simulink model "Battery_model_2D_Battery2"  (R2026a)
settings: Solver=VariableStepAuto  StopTime=10000
InitFcn:
  | %% Universal Parameters
  | 
  | Cycle_num = 1000; % number of cycles
  | 
  | Temp_state = 35;
  | 
  | 
  | SoC_state = 0.5;
  | 
  | OCV = [ 3.0025,3.4635,3.521,3.5618,3.6058,3.6426,3.6725,3.7049,3.7486,3.79951,3.8418,3.8738 ,3.9044,3.9448,3.9813,4.0222 ,4.0498,4.0658,4.0919,4.1359,4.2];
  | 
  | 
  | % Cn = 540; % As
  | Ru = 3.19; % KW^-1
  | Rc = 1.94; % KW^-1
  | Cc = 62.7; % JK^-1
  | Cs = 4.5;  % JK^-1
  | 
  | Ea = 31500;  % J * mol^-1
  | eta = 152.5; % unitless
  | Ic = 9000;   % [1/s] normalized current rate
  | Rg = 8.314;  % J / K / mol
  | z = 0.57;    % Ah power law exponent
  | 
  | 
  | 
  | %% Breakpoints
  | Temp = [5, 15, 25, 35, 45];
  | SoC  = [0, 0.05, 0.10, 0.15, 0.20, 0.25, 0.30, 0.35, 0.40, 0.45, 0.50, 0.55, 0.60, 0.65, 0.70, 0.75, 0.80, 0.85, 0.90, 0.95, 1.00];
  | 
  | %% ── CHARGING Parameters ──────────────────────────────────────────────────────
  | %% CHARGING Parameters
  | 
  | % --- R0 (charge) ---
  | R0_5_ch  = [0.10039366, 0.10039366, 0.10039366, 0.08528700, 0.07769698, 0.08283688, 0.11006698 ...
  |              0.11427069, 0.11402639, 0.11444591, 0.11423324, 0.11397462, 0.11400530, 0.11412006 ...
  |              0.11437022, 0.11469884, 0.11501972, 0.11491341, 0.11445199, 0.11423824, 0.11366247];
  | R0_15_ch  = [0.13171649, 0.13171649, 0.13171649, 0.11189655, 0.10193844, 0.10868199, 0.14440788 ...
  |              0.14992315, 0.14960263, 0.15015303, 0.14987401, 0.14953470, 0.14957496, 0.14972552 ...
  |              0.15005372, 0.15048488, 0.15090588, 0.15076639, 0.15016101, 0.14988057, 0.14912516];
  | R0_25_ch  = [0.15680534, 0.15680534, 0.15680534, 0.13321018, 0.12135528, 0.12938332, 0.17191415 ...
  |              0.17847994, 0.17809836, 0.17875361, 0.17842144, 0.17801751, 0.17806543, 0.17824467 ...
  |              0.17863539, 0.17914866, 0.17964985, 0.17948380, 0.17876310, 0.17842925, 0.17752995];
  | R0_35_ch  = [0.18293956, 0.18293956, 0.18293956, 0.15541187, 0.14158117, 0.15094720, 0.20056650 ...
  |              0.20822660, 0.20778142, 0.20854588, 0.20815835, 0.20768709, 0.20774300, 0.20795212 ...
  |              0.20840795, 0.20900677, 0.20959150, 0.20939777, 0.20855695, 0.20816746, 0.20711828];
  | R0_45_ch  = [0.20580701, 0.20580701, 0.20580701, 0.17483836, 0.15927881, 0.16981560, 0.22563732 ...
  |              0.23425492, 0.23375410, 0.23461411, 0.23417814, 0.23364798, 0.23371087, 0.23394613 ...
  |              0.23445894, 0.23513262, 0.23579043, 0.23557249, 0.23462657, 0.23418839, 0.23300807];
  | R0_ch = [R0_5_ch; R0_15_ch; R0_25_ch; R0_35_ch; R0_45_ch];
  | 
  | % --- R1 (charge) ---
  | R1_5_ch  = [0.04985788, 0.04985788, 0.05071229, 0.04160410, 0.03661133, 0.03925367, 0.05381930 ...
  |              0.05642225, 0.05603500, 0.05496214, 0.05471562, 0.05430091, 0.05382478, 0.05367572 ...
  |              0.05355262, 0.05341750, 0.05337771, 0.05361159, 0.05382278, 0.05411150, 0.05453301];
  | R1_15_ch  = [0.07380278, 0.07380278, 0.07506754, 0.06158502, 0.05419440, 0.05810577, 0.07966673 ...
  |              0.08351978, 0.08294655, 0.08135843, 0.08099351, 0.08037963, 0.07967483, 0.07945418 ...
  |              0.07927196, 0.07907196, 0.07901306, 0.07935925, 0.07967188, 0.08009926, 0.08072321];
  | R1_25_ch  = [0.09348353, 0.09348353, 0.09508555, 0.07800769, 0.06864625, 0.07360064, 0.10091119 ...
  |              0.10579172, 0.10506563, 0.10305401, 0.10259178, 0.10181420, 0.10092146, 0.10064197 ...
  | ... (+154 lines)
model workspace (MAT data in the model file):
  C_As = 150
  Cn = 150
  I_c = 1
  I_c_full_charged = 0.0333333333333
  Tc_state = 35.0044118318
  Ts_state = 35.0027406087
  V1_state = 0.00398713164124
  V2_state = 0.00927212980774
  V_cutoff = 3
  V_max = 4.2
  current_SoC = 0.996576803874
undefined symbols (not defined in the file): V1_ini
libraries: simulink x7
(part 2 of 2)

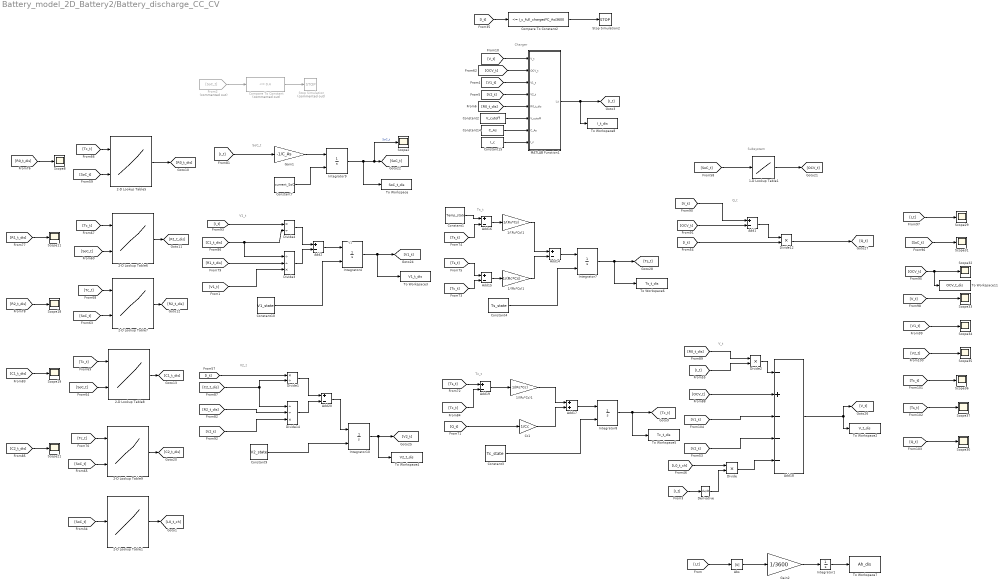
== system Battery_model_2D_Battery2/Battery_discharge_CC_CV ==
  note: Q_t
  note: V1
  note: SoC_t
  note: V1_t
  note: V2_t
  note: V_t
  note: Ts_t
  note: Tc_t
  note: Subsystem
  note: Charger
  1-D Lookup Table1 : Lookup_n-D  NumberOfTableDimensions=1  BreakpointsForDimension1=SoC  BreakpointsForDimension2=Temp  Table=OCV  InternalRulePriority=Speed  RndMeth=Simplest
  1/(Rc*Cc)1 : Gain  Gain=1/(Rc*Cc)
  1/(Rc*Cs)1 : Gain  Gain=1/(Rc*Cs)
  1/(Ru*Cs)1 : Gain  Gain=1/(Ru*Cs)
  2-D Lookup Table1 : Lookup_n-D  NumberOfTableDimensions=1  BreakpointsForDimension1=Temp  BreakpointsForDimension2=SoC  Table=C2_ch  InternalRulePriority=Speed  RndMeth=Simplest
  2-D Lookup Table5 : Lookup_n-D  BreakpointsForDimension1=Temp  BreakpointsForDimension2=SoC  Table=R0_dis  InternalRulePriority=Speed  RndMeth=Simplest
      settings: InputPortMap=u0,u1
  2-D Lookup Table6 : Lookup_n-D  BreakpointsForDimension1=Temp  BreakpointsForDimension2=SoC  Table=R1_dis  InternalRulePriority=Speed  RndMeth=Simplest
      settings: InputPortMap=u0,u1
  2-D Lookup Table7 : Lookup_n-D  BreakpointsForDimension1=Temp  BreakpointsForDimension2=SoC  Table=R2_dis  InternalRulePriority=Speed  RndMeth=Simplest
      settings: InputPortMap=u0,u1
  2-D Lookup Table8 : Lookup_n-D  BreakpointsForDimension1=Temp  BreakpointsForDimension2=SoC  Table=C1_dis  InternalRulePriority=Speed  RndMeth=Simplest
      settings: InputPortMap=u0,u1
  2-D Lookup Table9 : Lookup_n-D  BreakpointsForDimension1=Temp  BreakpointsForDimension2=SoC  Table=C2_dis  InternalRulePriority=Speed  RndMeth=Simplest
      settings: InputPortMap=u0,u1
  Abs : Abs  SaturateOnIntegerOverflow=off
  Add{1..2,14..16,19..20} (7 alike) : Sum  Inputs=+-
  Add17 : Sum
  Add18 : Sum  Inputs=-+---
  Cc1 : Gain  Gain=1/Cc
  Compare To Constant : simulink/Logic and Bit Operations/Compare To Constant  Commented=on  relop=<=  const=0.4  OutDataTypeStr=boolean
  Compare To Constant2 : simulink/Logic and Bit Operations/Compare To Constant  relop=<=  const=I_c_full_charged*C_As/3600  OutDataTypeStr=boolean
  Constant1 : Constant  Value=Temp_state
  Constant10 : Constant  Value=V1_state
  Constant14 : Constant  Value=C_As
  Constant15 : Constant  Value=I_c
  Constant2 : Constant  Value=V_cutoff
  Constant3 : Constant  Value=Tc_state
  Constant4 : Constant  Value=Ts_state
  Constant7 : Constant  Value=current_SoC
  Constant9 : Constant  Value=V2_state
  Derivative : Derivative
  Divide : Product  Inputs=**
  Divide1 : Product  Inputs=*/
  Divide12 : Product  Inputs=**
  Divide14 : Product  Inputs=//*
  Divide2 : Product  Inputs=**
  Divide3 : Product  Inputs=//*
  Divide4 : Product  Inputs=*/
  From2 : From  Commented=on  GotoTag=SoC_t
  Gain1 : Gain  Gain=-1/C_As
  Gain2 : Gain  Gain=1/3600
  Integrator1 : Integrator
  Integrator{4,7..8,10} (4 alike) : Integrator  InitialConditionSource=external
  Integrator9 : Integrator  InitialConditionSource=external  InitialCondition=V1_ini
  MATLAB Function1 : MATLAB Function  TreatAsAtomicUnit=on
  Scope{2,8,11,18..19,21,29..37} (15 alike) : Scope
      Scope11 settings: ActiveDisplayYMinimum=-0.125  ActiveDisplayYMaximum=1.125  DataLoggingVariableName=ScopeData7
      Scope18 settings: ActiveDisplayYMinimum=-0.125  ActiveDisplayYMaximum=1.125  DataLoggingVariableName=ScopeData8
      Scope19 settings: ActiveDisplayYMinimum=-0.125  ActiveDisplayYMaximum=1.125  DataLoggingVariableName=ScopeData9
      Scope2 settings: ActiveDisplayYMinimum=-1  ActiveDisplayYMaximum=1
      Scope21 settings: ActiveDisplayYMinimum=-0.125  ActiveDisplayYMaximum=1.125  DataLoggingVariableName=ScopeData10
      Scope29 settings: ActiveDisplayYMinimum=-0.013121  ActiveDisplayYMaximum=0.16808  DataLoggingVariableName=ScopeData15
      Scope30 settings: ActiveDisplayYMinimum=-0.17004  ActiveDisplayYMaximum=1.5304  DataLoggingVariableName=ScopeData23
      Scope31 settings: ActiveDisplayYMinimum=0.00061627  ActiveDisplayYMaximum=0.00083875  DataLoggingVariableName=ScopeData16
      Scope32 settings: ActiveDisplayYMinimum=2.011  ActiveDisplayYMaximum=4.011  DataLoggingVariableName=ScopeData17
      Scope33 settings: ActiveDisplayYMinimum=2.85  ActiveDisplayYMaximum=3.15  DataLoggingVariableName=ScopeData18
      Scope34 settings: ActiveDisplayYMinimum=0.0016856  ActiveDisplayYMaximum=0.0018374  DataLoggingVariableName=ScopeData19
      Scope35 settings: ActiveDisplayYMinimum=0.006752  ActiveDisplayYMaximum=0.008752  DataLoggingVariableName=ScopeData20
      Scope36 settings: ActiveDisplayYMinimum=-4.1824  ActiveDisplayYMaximum=42.6414  DataLoggingVariableName=ScopeData21
      Scope37 settings: ActiveDisplayYMinimum=2.2586  ActiveDisplayYMaximum=3.6824  DataLoggingVariableName=ScopeData22
      Scope8 settings: ActiveDisplayYMinimum=-0.125  ActiveDisplayYMaximum=1.125  DataLoggingVariableName=ScopeData6
  Stop Simulation : Stop  Commented=on
  Stop Simulation2 : Stop
  To Workspace : ToWorkspace  VariableName=SoC_t_dis  SampleTime=-1
      settings: Save2DSignal=2-D array (concatenate along first dimension)
  To Workspace11 : ToWorkspace  VariableName=OCV_t_dis  SaveFormat=Timeseries  SampleTime=-1
  To Workspace2 : ToWorkspace  VariableName=V_t_dis  SaveFormat=Timeseries  SampleTime=-1
  To Workspace3 : ToWorkspace  VariableName=V1_t_dis  SampleTime=-1
      settings: Save2DSignal=2-D array (concatenate along first dimension)
  To Workspace4 : ToWorkspace  VariableName=V2_t_dis  SampleTime=-1
      settings: Save2DSignal=2-D array (concatenate along first dimension)
  To Workspace5 : ToWorkspace  VariableName=Tc_t_dis  SampleTime=-1
      settings: Save2DSignal=2-D array (concatenate along first dimension)
  To Workspace6 : ToWorkspace  VariableName=Ts_t_dis  SampleTime=-1
      settings: Save2DSignal=2-D array (concatenate along first dimension)
  To Workspace7 : ToWorkspace  VariableName=Ah_dis  SampleTime=-1
      settings: Save2DSignal=2-D array (concatenate along first dimension)
  To Workspace8 : ToWorkspace  VariableName=I_t_dis  SaveFormat=Timeseries  SampleTime=-1
  wires:
  2-D Lookup Table9/1 -> [C2_t_dis]
  [SoC_t] -> 2-D Lookup Table9/2
  Add18/1 -> [V_t], To Workspace2/1
  [V2_t] -> Scope35/1
  Cc1/1 -> Add17/2
  Divide1/1 -> Add20/1
  1-D Lookup Table1/1 -> [OCV_t]
  [SoC_t] -> Scope31/1
  Gain1/1 -> Integrator9/1
  [Tc_t] -> 2-D Lookup Table5/1
  [OCV_t] -> Add18/2
  Integrator10/1 -> To Workspace4/1, [V2_t]
  1/(Rc*Cc)1/1 -> Add17/1
  [R0_t_dis] -> Scope8/1
  Integrator4/1 -> To Workspace3/1, [V1_t]
  Divide4/1 -> Add2/1
  [Ts_t] -> Add19/1
  [C2_t_dis] -> Divide14/1, Divide1/2
  [V2_t] -> Divide14/3
  1/(Ru*Cs)1/1 -> Add14/1
  [SoC_t] -> 2-D Lookup Table8/2
  Add17/1 -> Integrator8/1
  [Tc_t] -> Scope36/1
  Constant1/1 -> Add16/1
  Divide12/1 -> [Q_t]
  2-D Lookup Table8/1 -> [C1_t_dis]
  Integrator7/1 -> To Workspace6/1, [Ts_t]
  1/(Rc*Cs)1/1 -> Add14/2
  [R1_t_dis] -> Scope11/1
  [Ts_t] -> Add16/2
  [V1_t] -> Add18/3
  Add16/1 -> 1/(Ru*Cs)1/1
  Add1/1 -> Divide12/1
  [I_t] -> Scope29/1
  Divide14/1 -> Add20/2
  [R2_t_dis] -> Divide14/2
  [Q_t] -> Scope30/1
  Add14/1 -> Integrator7/1
  Add2/1 -> Integrator4/1
  [Tc_t] -> 2-D Lookup Table7/1
  [V1_t] -> Scope34/1
  2-D Lookup Table7/1 -> [R2_t_dis]
  2-D Lookup Table6/1 -> [R1_t_dis]
  [V2_t] -> Add18/4
  [SoC_t] -> 2-D Lookup Table6/2
  [R2_t_dis] -> Scope18/1
  [SoC_t] -> 2-D Lookup Table5/2
  2-D Lookup Table5/1 -> [R0_t_dis]
  [OCV_t] -> To Workspace11/1, Scope32/1
  [Q_t] -> Cc1/1
  Divide3/1 -> Add2/2
  [I_t] -> Divide12/2
  Add19/1 -> 1/(Rc*Cc)1/1
  Add20/1 -> Integrator10/1
  [C1_t_dis] -> Scope19/1
  Divide2/1 -> Add18/1
  Add15/1 -> 1/(Rc*Cs)1/1
  [R1_t_dis] -> Divide3/2
  [C1_t_dis] -> Divide4/2, Divide3/1
  Integrator9/1 -> To Workspace/1, Scope2/1, [SoC_t]  "SoC_t"
  [Tc_t] -> Add15/2
  [OCV_t] -> Add1/2
  [C2_t_dis] -> Scope21/1
  [Tc_t] -> 2-D Lookup Table8/1
  [V1_t] -> Divide3/3
  [Tc_t] -> 2-D Lookup Table9/1
  [Ts_t] -> Add15/1
  [Ts_t] -> Scope37/1
  [V_t] -> Scope33/1
  [SoC_t] -> 1-D Lookup Table1/1
  [SoC_t] -> 2-D Lookup Table7/2
  [Tc_t] -> 2-D Lookup Table6/1
  [R0_t_dis] -> Divide2/1
  Integrator8/1 -> To Workspace5/1, [Tc_t]
  [V_t] -> Add1/1
  Compare To Constant/1 -> Stop Simulation/1
  From2/1 -> Compare To Constant/1
  Constant10/1 -> Integrator4/2
  Constant4/1 -> Integrator7/2
  Constant9/1 -> Integrator10/2
  Constant3/1 -> Integrator8/2
  [I_t] -> Abs/1
  Integrator1/1 -> To Workspace7/1
  Gain2/1 -> Integrator1/1
  [I_t] -> Gain1/1
  MATLAB Function1/1(I_t) -> To Workspace8/1, [I_t]
  Constant2/1 -> MATLAB Function1/6(V_cutoff)
  Constant14/1 -> MATLAB Function1/7(C_As)
  [R0_t_dis] -> MATLAB Function1/5(R0_t_dis)
  Constant15/1 -> MATLAB Function1/8(I_c)
  [V_t] -> MATLAB Function1/1(V_t)
  [V2_t] -> MATLAB Function1/4(V2_t)
  [OCV_t] -> MATLAB Function1/2(OCV_t)
  [V1_t] -> MATLAB Function1/3(V1_t)
  [Tc_t] -> Add19/2
  [I_t] -> Compare To Constant2/1
  Compare To Constant2/1 -> Stop Simulation2/1
  Abs/1 -> Gain2/1
  [I_t] -> Divide4/1
  [I_t] -> Divide1/1
  [I_t] -> Divide2/2
  Constant7/1 -> Integrator9/2
  [SoC_t] -> 2-D Lookup Table1/1
  2-D Lookup Table1/1 -> [L0_t_ch]
  Derivative/1 -> Divide/2
  Divide/1 -> Add18/5
  [I_t] -> Derivative/1
  [L0_t_ch] -> Divide/1

== matlab function Battery_model_2D_Battery2/Battery_discharge_CC/MATLAB Function2 ==
  data: I_c input; I_t output; Cn input
function I_t = current_control(I_c,Cn)

    I_t = I_c*Cn/3600;
end

== matlab function Battery_model_2D_Battery2/Battery_charge_CC_CV/MATLAB Function1 ==
  data: I_t output; V_t input; OCV_t input; V1_t input; V2_t input; R0_t_ch input; V_max input; C_As input; I_c input
function I_t = current_control(V_t,OCV_t,V1_t,V2_t,R0_t_ch,V_max,C_As,I_c)
   
    if V_t < V_max
        I_t = I_c*C_As/3600;

    else
        I_t = (V_max - OCV_t - V1_t - V2_t)/R0_t_ch;
     
    end    
   
end

== matlab function Battery_model_2D_Battery2/Battery_charge_CC/MATLAB Function4 ==
  data: I_c input; I_t output; Cn input
function I_t = current_control(I_c,Cn)

    I_t = I_c*Cn/3600;
end

== matlab function Battery_model_2D_Battery2/Battery_discharge_CC_CV/MATLAB Function1 ==
  data: I_t output; V_t input; OCV_t input; V1_t input; V2_t input; R0_t_dis input; V_cutoff input; C_As input; I_c input
function I_t = current_control(V_t,OCV_t,V1_t,V2_t,R0_t_dis,V_cutoff,C_As,I_c)
   
    if V_t > V_cutoff
        I_t = I_c*C_As/3600;

    else
        I_t = (-V_cutoff + OCV_t - V1_t - V2_t)/R0_t_dis;
     
    end    
   
end
